simulink model "HDLMultipleClock"  (R2024a)
settings: Solver=FixedStepDiscrete  StartTime=0.0  StopTime=stopTime  RelTol=1e-3
values from neighbouring files (symbols this model uses):
  fs = 100e6    (= 100000000)    [testMultipleClock.m]
libraries: dspsrcs4 x2, hdlsllib x2
settings Model: DataTypeOverride=Off  Creator=cotti  LastModifiedBy=cotti
settings OptimizationCC: BlockReduction=off  ConditionallyExecuteInputs=off  DefaultParameterBehavior=Inlined  InheritOutputTypeSmallerThanSingle=on
settings DebuggingCC: AlgebraicLoopMsg=error  ArtificialAlgebraicLoopMsg=error  SingleTaskRateTransMsg=error  UnconnectedInputMsg=warning  UnconnectedOutputMsg=warning  UnconnectedLineMsg=warning
settings HardwareCC: ProdBitPerPointer=32  ProdBitPerSizeT=32  ProdBitPerPtrDiffT=32  ProdLargestAtomicFloat=None  ProdIntDivRoundTo=Undefined  ProdEndianess=Unspecified  ProdWordSize=32  ProdHWDeviceType=ASIC/FPGA->ASIC/FPGA  TargetBitPerLong=64  TargetBitPerPointer=64  TargetBitPerSizeT=64  TargetBitPerPtrDiffT=64  TargetLongLongMode=on  TargetIntDivRoundTo=Zero  TargetEndianess=LittleEndian  TargetWordSize=64  TargetHWDeviceType=Custom Processor->MATLAB Host Computer  ProdEqTarget=off

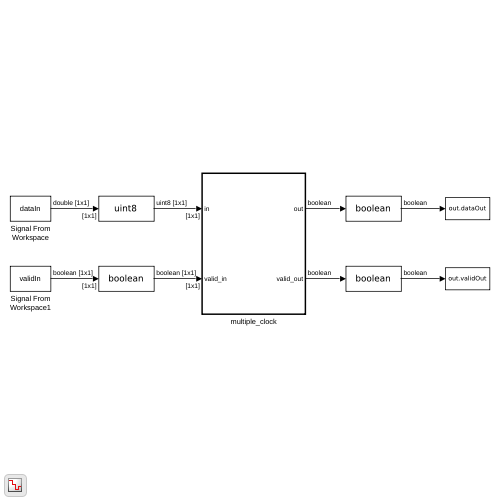
[thumbnail: Simulink's stored preview of the top-level diagram]
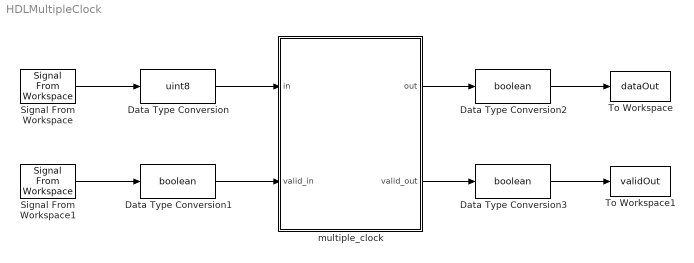
== system HDLMultipleClock ==
  Data Type Conversion : DataTypeConversion  OutDataTypeStr=uint8  SaturateOnIntegerOverflow=off  RndMeth=Floor
  Data Type Conversion1 : DataTypeConversion  OutDataTypeStr=boolean  SaturateOnIntegerOverflow=off  RndMeth=Floor
  Data Type Conversion2 : DataTypeConversion  OutDataTypeStr=boolean  SaturateOnIntegerOverflow=off  RndMeth=Floor
  Data Type Conversion3 : DataTypeConversion  OutDataTypeStr=boolean  SaturateOnIntegerOverflow=off  RndMeth=Floor
  Signal From Workspace : dspsrcs4/Signal From Workspace  X=dataIn  Ts=8/fs  nsamps=1  OutputAfterFinalValue=Setting to zero  ignoreOrWarnInputAndFrameLengths=off  OutputFrames=off
  Signal From Workspace1 : dspsrcs4/Signal From Workspace  X=validIn  Ts=8/fs  nsamps=1  OutputAfterFinalValue=Setting to zero  ignoreOrWarnInputAndFrameLengths=off  OutputFrames=off
  To Workspace : ToWorkspace  VariableName=dataOut  SampleTime=1/fs
      settings: Save2DSignal=2-D array (concatenate along first dimension)
  To Workspace1 : ToWorkspace  VariableName=validOut  SampleTime=1/fs
      settings: Save2DSignal=2-D array (concatenate along first dimension)
  multiple_clock : Subsystem  TreatAsAtomicUnit=on
  wires:
  multiple_clock/1(out) -> Data Type Conversion2/1
  Signal From Workspace/1 -> Data Type Conversion/1
  Signal From Workspace1/1 -> Data Type Conversion1/1
  multiple_clock/2(valid_out) -> Data Type Conversion3/1
  Data Type Conversion/1 -> multiple_clock/1(in)
  Data Type Conversion1/1 -> multiple_clock/2(valid_in)
  Data Type Conversion2/1 -> To Workspace/1
  Data Type Conversion3/1 -> To Workspace1/1

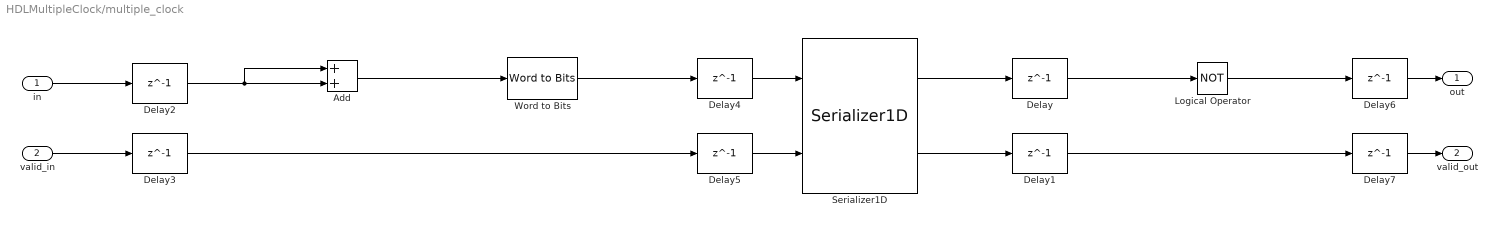
== system HDLMultipleClock/multiple_clock ==
  in : Inport
  valid_in : Inport  Port=2
  Add : Sum  OutDataTypeStr=uint8
  Delay{,1..7} (8 alike) : Delay  DelayLength=1  InitialCondition=0  UseCircularBuffer=on
  Logical Operator : Logic  Operator=NOT  AllPortsSameDT=off  OutDataTypeStr=boolean
  Serializer1D : hdlsllib/HDL Operations/Serializer1D  Ratio=8  IdleCycles=0  validIn=on  startOut=off  validOut=on  inputDataDimensions=-1  inputSampleTime=-1  inputSignalType=auto
  Word to Bits : hdlsllib/Logic and Bit Operations/Word to Bits  maxWordLength=8
  out : Outport
  valid_out : Outport  Port=2  VectorParamsAs1DForOutWhenUnconnected=off
  wires:
  Serializer1D/1 -> Delay/1
  in/1 -> Delay2/1
  Serializer1D/2 -> Delay1/1
  valid_in/1 -> Delay3/1
  Delay1/1 -> Delay7/1
  Word to Bits/1 -> Delay4/1
  Delay3/1 -> Delay5/1
  Delay4/1 -> Serializer1D/1
  Delay5/1 -> Serializer1D/2
  Delay6/1 -> out/1
  Delay7/1 -> valid_out/1
  Delay/1 -> Logical Operator/1
  Logical Operator/1 -> Delay6/1
  Delay2/1 -> Add/2, Add/1
  Add/1 -> Word to Bits/1
